simulink model "ex_2_20_simul"  (R2025a)
settings: Solver=VariableStepAuto  StartTime=0.0  StopTime=10.0  RelTol=1e-3
libraries: dspsrcs4 x1
settings Model: Creator=konstantin  LastModifiedBy=konstantin

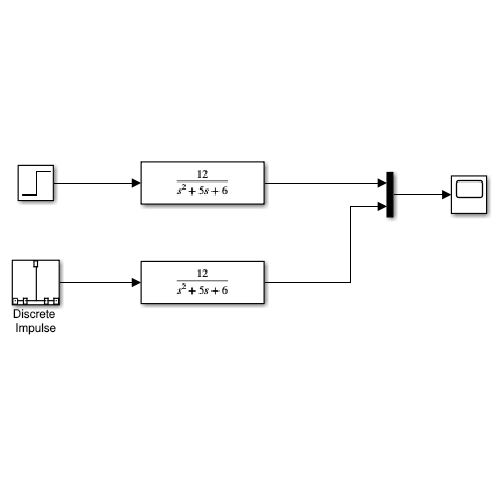
[thumbnail: Simulink's stored preview of the top-level diagram]
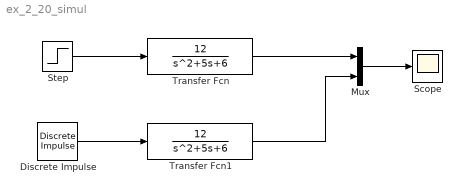
== system ex_2_20_simul ==
  Discrete Impulse : dspsrcs4/Discrete  Impulse  Delay=0  SampleTime=1.5  FrameSample=1  OutputFrames=off  dataType=double  isSigned=on  wordLen=16  udDataType=sfix(16)  fracBitsMode=Best precision  numFracBits=15  OutDataTypeStr=double  LastOutDataTypeStr=double
  Mux : Mux  Inputs=2
  Scope : Scope
      settings: ActiveDisplayYMinimum=-0.51883154435416756  ActiveDisplayYMaximum=2.376014773226967
  Step : Step  Time=0  SampleTime=0
  Transfer Fcn : TransferFcn  Numerator=[12]  Denominator=[1 5 6]
  Transfer Fcn1 : TransferFcn  Numerator=[12]  Denominator=[1 5 6]
  wires:
  Step/1 -> Transfer Fcn/1
  Discrete Impulse/1 -> Transfer Fcn1/1
  Transfer Fcn1/1 -> Mux/2
  Transfer Fcn/1 -> Mux/1
  Mux/1 -> Scope/1
